simulink model "Model_TranslationEngine64"  (R2022b)
settings: Solver=FixedStepDiscrete  StartTime=0.0  StopTime=5  RelTol=1e-3  EnableMultiTasking=on
InitFcn:
  | % Initialize model
  | ModelSettings=BTConfig.GetModelSettings();
  | 
  | ModelSettings.Validate();
  | 
  | ModelInit;
  | 
  | 
  | % load library data
  | GainLibrary_data;
  | % Load saved values from partition process
  | CapturedConstMask.LoadMapFromFile(bdroot)
StartFcn:
  | % make sure all the simulated RTC requests are found
  | %RTC_SIM_OBJ.ValidateREQs();
undefined symbols (not defined in the file or in its folder): AA, BPLP, Column, NumHFRefBPF, NumHFRefLPF, NumMusicChannels, Row, VolumeMuteConfig
libraries: TuneVar x925, TOP x490, FeaturePath x111, CapturedConstLib x52
(part 32 of 34)

== matlab function Model_TranslationEngine64/ModelPreAmp/DecRate/Medusa5H1/MedusaHoligram/Medusa5H1 Part 3/On/Full-rate Mixer/Full-Rate Mixer with CAE & Fade Ramper/Fade Tuning/Downmix Weights Left/Trivial Translation ==
  data: TOP output size=[MedusaFRMConfig.LR_out MedusaFRMConfig.LR_in]; downmix_wts_Left input; MedusaFRMConfig parameter; TOP_CAE output size=[MedusaFRMConfig.LR_out MedusaFRMConfig.NumTailComp.LR]
  events: trigger input FUNCTION_CALL_EVENT
function [TOP,TOP_CAE]  = fcn(downmix_wts_Left, MedusaFRMConfig)
%#codegen
numLRIn = MedusaFRMConfig.LR_in;
NumCAEWeights = MedusaFRMConfig.NumTailComp.LR;

NumRows = MedusaFRMConfig.LR_out;
NumColumns = numLRIn + NumCAEWeights;
if(~ MedusaFRMConfig.includeCAE)
    NumColumns = numLRIn;
end

% Checks if the parameter satisfies dimensionality requirements
if(downmix_wts_Left.Size(1) ~= NumRows || downmix_wts_Left.Size(2) ~= NumColumns)
    TranslateError('The parameter ''medusa_frm_downmix_left'' must be a matrix consisting of %d rows and %d columns.', NumRows, NumColumns);
end

% Checks if the parameter values follow bound requirements
checkValues = (downmix_wts_Left.Value < 0);
if(sum(sum(checkValues)))          % Results in 0 if all values in the matrix respect the bound requirements
    TranslateError('The weights in ''medusa_frm_downmix_left'' must be greater than or equal to 0.');
end

% Assigning the parameter values to respective tuneTOPS
TOP = downmix_wts_Left.Value(:, 1:numLRIn);
if(~ MedusaFRMConfig.includeCAE)
    TOP_CAE = zeros(NumRows, NumCAEWeights);
else
    TOP_CAE = downmix_wts_Left.Value(:, numLRIn+1:end);
end

end

== matlab function Model_TranslationEngine64/ModelPreAmp/DecRate/Medusa5H1/MedusaHoligram/Medusa5H1 Part 3/On/Full-rate Mixer/Full-Rate Mixer with CAE & Fade Ramper/Fade Tuning/Downmix Weights Right/Trivial Translation ==
  data: TOP output size=[MedusaFRMConfig.LR_out MedusaFRMConfig.LR_in]; downmix_wts_Right input; MedusaFRMConfig parameter; TOP_CAE output size=[MedusaFRMConfig.LR_out MedusaFRMConfig.NumTailComp.LR]
  events: trigger input FUNCTION_CALL_EVENT
function [TOP,TOP_CAE]  = fcn(downmix_wts_Right, MedusaFRMConfig)
%#codegen
numLRIn = MedusaFRMConfig.LR_in;
NumCAEWeights = MedusaFRMConfig.NumTailComp.LR;

NumRows = MedusaFRMConfig.LR_out;
NumColumns = numLRIn + NumCAEWeights;
if(~ MedusaFRMConfig.includeCAE)
    NumColumns = numLRIn;
end

% Checks if the parameter satisfies dimensionality requirements
if(downmix_wts_Right.Size(1) ~= NumRows || downmix_wts_Right.Size(2) ~= NumColumns)
    TranslateError('The parameter ''medusa_frm_downmix_right'' must be a matrix consisting of %d rows and %d columns.', NumRows, NumColumns);
end

% Checks if the parameter values follow bound requirements
checkValues = (downmix_wts_Right.Value < 0);
if(sum(sum(checkValues)))          % Results in 0 if all values in the matrix respect the bound requirements
    TranslateError('The weights in ''medusa_frm_downmix_right'' must be greater than or equal to 0.');
end

% Assigning the parameter values to respective tuneTOPS
TOP = downmix_wts_Right.Value(:, 1:numLRIn);
if(~ MedusaFRMConfig.includeCAE)
    TOP_CAE = zeros(NumRows, NumCAEWeights);
else
    TOP_CAE = downmix_wts_Right.Value(:, numLRIn+1:end);
end

end

== matlab function Model_TranslationEngine64/ModelPreAmp/DecRate/Medusa5H1/MedusaHoligram/Medusa5H1 Part 3/On/Full-rate Mixer/Full-Rate Mixer with CAE & Fade Ramper/Fade Tuning/Forward Downmix Threshold/Trivial Translation ==
  data: TOP output; ForwardDownmixThreshold input
  events: trigger input FUNCTION_CALL_EVENT
function TOP  = fcn(ForwardDownmixThreshold)
%#codegen
% Checks if the parameter satisfies dimensionality requirements
if(numel(ForwardDownmixThreshold.Value) ~= 1)
   TranslateError('The parameter ''medusa_forward_downmix_threshold'' must be single dimensional.'); 
end

% Checks if the parameter value follows bound requirements
if((ForwardDownmixThreshold.Value < 0) || (ForwardDownmixThreshold.Value > 1))
   TranslateError('The value of ''medusa_forward_downmix_threshold'' must be between 0 and 1.'); 
end

TOP = ForwardDownmixThreshold.Value;

end

== matlab function Model_TranslationEngine64/ModelPreAmp/DecRate/Medusa5H1/MedusaHoligram/Medusa5H1 Part 3/On/Full-rate Mixer/Full-Rate Mixer with CAE & Fade Ramper/Fade Tuning/Foward Downmix Max/Trivial Translation ==
  data: TOP output; ForwardDownmixMax input
  events: trigger input FUNCTION_CALL_EVENT
function TOP  = fcn(ForwardDownmixMax)
%#codegen
% Checks if the parameter satisfies dimensionality requirements
if(numel(ForwardDownmixMax.Value) ~= 1)
   TranslateError('The parameter ''medusa_forward_downmix_max'' must be single dimensional.'); 
end

% Checks if the parameter value follows bound requirements
if((ForwardDownmixMax.Value < 0) || (ForwardDownmixMax.Value > 1))
   TranslateError('The value of ''medusa_forward_downmix_max'' must be between 0 and 1.'); 
end

TOP = ForwardDownmixMax.Value;

end

== matlab function Model_TranslationEngine64/ModelPreAmp/DecRate/AudioPilot35/Audiopilot_3_5/NoiseEstimationVariant/RegularNoiseEstimation/HFNoiseEstimatorCoh/PreProcessing/Bandpass or Lowpass Filter/InnerLink/PoolIirTunableWithReset/Translation ==
  data: RawSOS input; NumStages input; PoolNumStages output; PoolCoeffs output; MaxNumStages parameter; VariantUint8 parameter; NumChannels input
  events: trigger input FUNCTION_CALL_EVENT
function [PoolNumStages, PoolCoeffs] = pooliirTranslation(RawSOS, NumStages, MaxNumStages, VariantUint8,  NumChannels)
%#codegen

% Translation from raw SOS for pool SOS

% Some build time sanity size checking before calling the translation
if numel(NumStages.Value) ~= NumChannels
    error('Size of num stages has to match number of input channels')
end

if RawSOS.Size(2) ~= 6
    error ('Coefficient pool matrix must have 6 columns')
end

[PoolNumStages, PoolCoeffs] = poolIirTranslation(RawSOS, NumStages, MaxNumStages, VariantUint8);

% VariantStr = char(VariantUint8);
% switch (VariantStr)
%     case {"Generic","SharcPlusCore"}
%         % These variants order biquad coefficients in a compacted form
%         [PoolNumStages, PoolCoeffs] = pooliirTranslationFcn(RawSOS, NumStages, MaxNumStages);
%     case {"SharcPlusAccelGul","SharcPlusAccelGxp"}
%         % These variants order biquad coefficients for the ADI accelerator
%         [PoolNumStages, PoolCoeffs] = pooliirAccelTranslationFcn(RawSOS, NumStages, MaxNumStages);
%     case{"Hexagon"}
%         % Hexagon specific order for biquad coefficients 
%         [PoolNumStages, PoolCoeffs] = PoolIirHexagonTranslationFcn(RawSOS, NumStages, MaxNumStages);
%     case{"ArmNeonV7V8"}
%         [PoolNumStages, PoolCoeffs] = PoolIirArmNeonV7V8TranslationFcn(RawSOS, NumStages, MaxNumStages);
%     otherwise
%         % This is a build-time error, not a translation error. The
%         % selected build-time variant is not supported for translation
%         error('Invalid implementation type: [%s]', VariantStr);
% end

end

== matlab function Model_TranslationEngine64/ModelPreAmp/DecRate/Medusa5H1/MedusaHoligram/Medusa5H1 Part 3/On/Full-rate Mixer/Full-Rate Mixer with CAE & Fade Ramper/SLC Tuning/Detent Level CS/Trivial Translation ==
  data: TOP output size=[MedusaFRMConfig.CS_out MedusaFRMConfig.CS_in]; detentGain_CS input; MedusaFRMConfig parameter; TOP_CAE output size=[MedusaFRMConfig.CS_out MedusaFRMConfig.NumTailComp.CS]
  events: trigger input FUNCTION_CALL_EVENT
function [TOP, TOP_CAE]  = fcn(detentGain_CS, MedusaFRMConfig)
%#codegen
numCSIn = MedusaFRMConfig.CS_in;
NumCAEWeights = MedusaFRMConfig.NumTailComp.CS;

NumRows = MedusaFRMConfig.CS_out;
NumColumns = numCSIn + NumCAEWeights;
if(~ MedusaFRMConfig.includeCAE)
    NumColumns = numCSIn;
end

% Checks if the parameter satisfies dimensionality requirements
if(detentGain_CS.Size(1) ~= NumRows || detentGain_CS.Size(2) ~= NumColumns)
    TranslateError('The parameter ''medusa_frm_cs_detent'' must be a matrix consisting of %d rows and %d columns.', NumRows, NumColumns);
end

% Checks if the parameter values follow bound requirements
checkValues = (detentGain_CS.Value < 0);    
if(sum(sum(checkValues)))       % Results in 0 if all values in the matrix respect the bound requirements
    TranslateError('The weights in ''medusa_frm_cs_detent'' must be greater than or equal to 0.');
end

% Assigning the parameter values to respective tuneTOPS
TOP = detentGain_CS.Value(:, 1:numCSIn);
if(~ MedusaFRMConfig.includeCAE)
    TOP_CAE = zeros(NumRows, NumCAEWeights);
else
    TOP_CAE = detentGain_CS.Value(:, numCSIn+1:end);
end

end

== matlab function Model_TranslationEngine64/ModelPreAmp/DecRate/Medusa5H1/MedusaHoligram/Medusa5H1 Part 3/On/Full-rate Mixer/Full-Rate Mixer with CAE & Fade Ramper/SLC Tuning/Detent Level Left/Trivial Translation ==
  data: TOP output size=[MedusaFRMConfig.LR_out MedusaFRMConfig.LR_in]; detentGain_Left input; MedusaFRMConfig parameter; TOP_CAE output size=[MedusaFRMConfig.LR_out MedusaFRMConfig.NumTailComp.LR]
  events: trigger input FUNCTION_CALL_EVENT
function [TOP, TOP_CAE]  = fcn(detentGain_Left, MedusaFRMConfig)
%#codegen
numLRIn = MedusaFRMConfig.LR_in;
NumCAEWeights = MedusaFRMConfig.NumTailComp.LR;

NumRows = MedusaFRMConfig.LR_out;
NumColumns = numLRIn + NumCAEWeights;
if(~ MedusaFRMConfig.includeCAE)
    NumColumns = numLRIn;
end

% Checks if the parameter satisfies dimensionality requirements
if(detentGain_Left.Size(1) ~= NumRows || detentGain_Left.Size(2) ~= NumColumns)
    TranslateError('The parameter ''medusa_frm_left_detent'' must be a matrix consisting of %d rows and %d columns.', NumRows, NumColumns);
end

% Checks if the parameter values follow bound requirements
checkValues = (detentGain_Left.Value < 0);    
if(sum(sum(checkValues)))       % Results in 0 if all values in the matrix respect the bound requirements
    TranslateError('The weights in ''medusa_frm_left_detent'' must be greater than or equal to 0.');
end

% Assigning the parameter values to respective tuneTOPS
TOP = detentGain_Left.Value(:, 1:numLRIn);
if(~ MedusaFRMConfig.includeCAE)
    TOP_CAE = zeros(NumRows, NumCAEWeights);
else
    TOP_CAE = detentGain_Left.Value(:, numLRIn+1:end);
end

end

== matlab function Model_TranslationEngine64/ModelPreAmp/DecRate/Medusa5H1/MedusaHoligram/Medusa5H1 Part 3/On/Full-rate Mixer/Full-Rate Mixer with CAE & Fade Ramper/SLC Tuning/Detent Level Right/Trivial Translation ==
  data: TOP output size=[MedusaFRMConfig.LR_out MedusaFRMConfig.LR_in]; detentGain_Right input; MedusaFRMConfig parameter; TOP_CAE output size=[MedusaFRMConfig.LR_out MedusaFRMConfig.NumTailComp.LR]
  events: trigger input FUNCTION_CALL_EVENT
function [TOP, TOP_CAE]  = fcn(detentGain_Right, MedusaFRMConfig)
%#codegen
numLRIn = MedusaFRMConfig.LR_in;
NumCAEWeights = MedusaFRMConfig.NumTailComp.LR;

NumRows = MedusaFRMConfig.LR_out;
NumColumns = numLRIn + NumCAEWeights;
if(~ MedusaFRMConfig.includeCAE)
    NumColumns = numLRIn;
end

% Checks if the parameter satisfies dimensionality requirements
if(detentGain_Right.Size(1) ~= NumRows || detentGain_Right.Size(2) ~= NumColumns)
    TranslateError('The parameter ''medusa_frm_right_detent'' must be a matrix consisting of %d rows and %d columns.', NumRows, NumColumns);
end

% Checks if the parameter values follow bound requirements
checkValues = (detentGain_Right.Value < 0);    
if(sum(sum(checkValues)))       % Results in 0 if all values in the matrix respect the bound requirements
    TranslateError('The weights in ''medusa_frm_right_detent'' must be greater than or equal to 0.');
end

% Assigning the parameter values to respective tuneTOPS
TOP = detentGain_Right.Value(:, 1:numLRIn);
if(~ MedusaFRMConfig.includeCAE)
    TOP_CAE = zeros(NumRows, NumCAEWeights);
else
    TOP_CAE = detentGain_Right.Value(:, numLRIn+1:end);
end

end

== matlab function Model_TranslationEngine64/ModelPreAmp/DecRate/Medusa5H1/MedusaHoligram/Medusa5H1 Part 3/On/Full-rate Mixer/Full-Rate Mixer with CAE & Fade Ramper/SLC Tuning/Interpolation Method/Trivial Translation ==
  data: TOP output; interpolationMethod input
  events: trigger input FUNCTION_CALL_EVENT
function TOP  = fcn(interpolationMethod)
%#codegen
% Checks if the parameter satisfies dimensionality requirements
if(numel(interpolationMethod.Value) ~= 1)
   TranslateError('The parameter ''medusa_surround_db_interpolation'' must be single dimensional.'); 
end

% Checks if the parameter value follows bound requirements
if((interpolationMethod.Value ~= 0) && (interpolationMethod.Value ~= 1))
   TranslateError('The value of ''medusa_surround_db_interpolation'' must be either 0 (for linear interpolation) or 1 (for dB-linear interpolation).'); 
end

TOP = interpolationMethod.Value;

end

== matlab function Model_TranslationEngine64/ModelPreAmp/DecRate/Medusa5H1/MedusaHoligram/Medusa5H1 Part 3/On/Full-rate Mixer/Full-Rate Mixer with CAE & Fade Ramper/SLC Tuning/Max Level CS/Trivial Translation ==
  data: TOP output size=[MedusaFRMConfig.CS_out MedusaFRMConfig.CS_in]; maxGain_CS input; MedusaFRMConfig parameter; TOP_CAE output size=[MedusaFRMConfig.CS_out MedusaFRMConfig.NumTailComp.CS]
  events: trigger input FUNCTION_CALL_EVENT
function [TOP, TOP_CAE] = fcn(maxGain_CS, MedusaFRMConfig)
%#codegen
numCSIn = MedusaFRMConfig.CS_in;
NumCAEWeights = MedusaFRMConfig.NumTailComp.CS;

NumRows = MedusaFRMConfig.CS_out;
NumColumns = numCSIn + NumCAEWeights;
if(~ MedusaFRMConfig.includeCAE)
    NumColumns = numCSIn;
end

% Checks if the parameter satisfies dimensionality requirements
if(maxGain_CS.Size(1) ~= NumRows || maxGain_CS.Size(2) ~= NumColumns)
    TranslateError('The parameter ''medusa_frm_cs_max'' must be a matrix consisting of %d rows and %d columns.', NumRows, NumColumns);
end

% Checks if the parameter values follow bound requirements
checkValues = (maxGain_CS.Value < 0);
if(sum(sum(checkValues)))          % Results in 0 if all values in the matrix respect the bound requirements
    TranslateError('The weights in ''medusa_frm_cs_max'' must be greater than or equal to 0.');
end

% Assigning the parameter values to respective tuneTOPS
TOP = maxGain_CS.Value(:, 1:numCSIn);
if(~ MedusaFRMConfig.includeCAE)
    TOP_CAE = zeros(NumRows, NumCAEWeights);
else
    TOP_CAE = maxGain_CS.Value(:, numCSIn+1:end);
end

end

== matlab function Model_TranslationEngine64/ModelPreAmp/DecRate/Medusa5H1/MedusaHoligram/Medusa5H1 Part 3/On/Full-rate Mixer/Full-Rate Mixer with CAE & Fade Ramper/SLC Tuning/Max Level Left/Trivial Translation ==
  data: TOP output size=[MedusaFRMConfig.LR_out MedusaFRMConfig.LR_in]; maxGain_Left input; MedusaFRMConfig parameter; TOP_CAE output size=[MedusaFRMConfig.LR_out MedusaFRMConfig.NumTailComp.LR]
  events: trigger input FUNCTION_CALL_EVENT
function [TOP, TOP_CAE]  = fcn(maxGain_Left, MedusaFRMConfig)
%#codegen
numLRIn = MedusaFRMConfig.LR_in;
NumCAEWeights = MedusaFRMConfig.NumTailComp.LR;

NumRows = MedusaFRMConfig.LR_out;
NumColumns = numLRIn + NumCAEWeights;
if(~ MedusaFRMConfig.includeCAE)
    NumColumns = numLRIn;
end

% Checks if the parameter satisfies dimensionality requirements
if(maxGain_Left.Size(1) ~= NumRows || maxGain_Left.Size(2) ~= NumColumns)
    TranslateError('The parameter ''medusa_frm_left_max'' must be a matrix consisting of %d rows and %d columns.', NumRows, NumColumns);
end

% Checks if the parameter values follow bound requirements
checkValues = (maxGain_Left.Value < 0);
if(sum(sum(checkValues)))          % Results in 0 if all values in the matrix respect the bound requirements
    TranslateError('The weights in ''medusa_frm_left_max'' must be greater than or equal to 0.');
end

% Assigning the parameter values to respective tuneTOPS
TOP = maxGain_Left.Value(:, 1:numLRIn);
if(~ MedusaFRMConfig.includeCAE)
    TOP_CAE = zeros(NumRows, NumCAEWeights);
else
    TOP_CAE = maxGain_Left.Value(:, numLRIn+1:end);
end

end

== matlab function Model_TranslationEngine64/ModelPreAmp/DecRate/Medusa5H1/MedusaHoligram/Medusa5H1 Part 3/On/Full-rate Mixer/Full-Rate Mixer with CAE & Fade Ramper/SLC Tuning/Max Level Right/Trivial Translation ==
  data: TOP output size=[MedusaFRMConfig.LR_out MedusaFRMConfig.LR_in]; maxGain_Right input; MedusaFRMConfig parameter; TOP_CAE output size=[MedusaFRMConfig.LR_out MedusaFRMConfig.NumTailComp.LR]
  events: trigger input FUNCTION_CALL_EVENT
function [TOP, TOP_CAE]  = fcn(maxGain_Right, MedusaFRMConfig)
%#codegen
numLRIn = MedusaFRMConfig.LR_in;
NumCAEWeights = MedusaFRMConfig.NumTailComp.LR;

NumRows = MedusaFRMConfig.LR_out;
NumColumns = numLRIn + NumCAEWeights;
if(~ MedusaFRMConfig.includeCAE)
    NumColumns = numLRIn;
end

% Checks if the parameter satisfies dimensionality requirements
if(maxGain_Right.Size(1) ~= NumRows || maxGain_Right.Size(2) ~= NumColumns)
    TranslateError('The parameter ''medusa_frm_right_max'' must be a matrix consisting of %d rows and %d columns.', NumRows, NumColumns);
end

% Checks if the parameter values follow bound requirements
checkValues = (maxGain_Right.Value < 0);
if(sum(sum(checkValues)))          % Results in 0 if all values in the matrix respect the bound requirements
    TranslateError('The weights in ''medusa_frm_right_max'' must be greater than or equal to 0.');
end

% Assigning the parameter values to respective tuneTOPS
TOP = maxGain_Right.Value(:, 1:numLRIn);
if(~ MedusaFRMConfig.includeCAE)
    TOP_CAE = zeros(NumRows, NumCAEWeights);
else
    TOP_CAE = maxGain_Right.Value(:, numLRIn+1:end);
end

end

== matlab function Model_TranslationEngine64/ModelPreAmp/DecRate/Medusa5H1/MedusaHoligram/Medusa5H1 Part 3/On/Full-rate Mixer/Full-Rate Mixer with CAE & Fade Ramper/SLC Tuning/Min Level CS/Trivial Translation ==
  data: TOP output size=[MedusaFRMConfig.CS_out MedusaFRMConfig.CS_in]; minGain_CS input; MedusaFRMConfig parameter; TOP_CAE output size=[MedusaFRMConfig.CS_out MedusaFRMConfig.NumTailComp.CS]
  events: trigger input FUNCTION_CALL_EVENT
function [TOP, TOP_CAE]  = fcn(minGain_CS, MedusaFRMConfig)
%#codegen
numCSIn = MedusaFRMConfig.CS_in;
NumCAEWeights = MedusaFRMConfig.NumTailComp.CS;

NumRows = MedusaFRMConfig.CS_out;
NumColumns = numCSIn + NumCAEWeights;
if(~ MedusaFRMConfig.includeCAE)
    NumColumns = numCSIn;
end

% Checks if the parameter satisfies dimensionality requirements
if(minGain_CS.Size(1) ~= NumRows || minGain_CS.Size(2) ~= NumColumns)
    TranslateError('The parameter ''medusa_frm_cs_min'' must be a matrix consisting of %d rows and %d columns.', NumRows, NumColumns);
end

% Checks if the parameter values follow bound requirements
checkValues = (minGain_CS.Value < 0);
if(sum(sum(checkValues)))          % Results in 0 if all values in the matrix respect the bound requirements
    TranslateError('The weights in ''medusa_frm_cs_min'' must be greater than or equal to 0.');
end

% Assigning the parameter values to respective tuneTOPS
TOP = minGain_CS.Value(:, 1:numCSIn);
if(~ MedusaFRMConfig.includeCAE)
    TOP_CAE = zeros(NumRows, NumCAEWeights);
else
    TOP_CAE = minGain_CS.Value(:, numCSIn+1:end);
end

end

== matlab function Model_TranslationEngine64/ModelPreAmp/DecRate/Medusa5H1/MedusaHoligram/Medusa5H1 Part 3/On/Full-rate Mixer/Full-Rate Mixer with CAE & Fade Ramper/SLC Tuning/Min Level Left/Trivial Translation ==
  data: TOP output size=[MedusaFRMConfig.LR_out MedusaFRMConfig.LR_in]; minGain_Left input; MedusaFRMConfig parameter; TOP_CAE output size=[MedusaFRMConfig.LR_out MedusaFRMConfig.NumTailComp.LR]
  events: trigger input FUNCTION_CALL_EVENT
function [TOP, TOP_CAE]  = fcn(minGain_Left, MedusaFRMConfig)
%#codegen
numLRIn = MedusaFRMConfig.LR_in;
NumCAEWeights = MedusaFRMConfig.NumTailComp.LR;

NumRows = MedusaFRMConfig.LR_out;
NumColumns = numLRIn + NumCAEWeights;
if(~ MedusaFRMConfig.includeCAE)
    NumColumns = numLRIn;
end

% Checks if the parameter satisfies dimensionality requirements
if(minGain_Left.Size(1) ~= NumRows || minGain_Left.Size(2) ~= NumColumns)
    TranslateError('The parameter ''medusa_frm_left_min'' must be a matrix consisting of %d rows and %d columns.', NumRows, NumColumns);
end

% Checks if the parameter values follow bound requirements
checkValues = (minGain_Left.Value < 0);
if(sum(sum(checkValues)))          % Results in 0 if all values in the matrix respect the bound requirements
    TranslateError('The weights in ''medusa_frm_left_min'' must be greater than or equal to 0.');
end

% Assigning the parameter values to respective tuneTOPS
TOP = minGain_Left.Value(:, 1:numLRIn);
if(~ MedusaFRMConfig.includeCAE)
    TOP_CAE = zeros(NumRows, NumCAEWeights);
else
    TOP_CAE = minGain_Left.Value(:, numLRIn+1:end);
end

end

== matlab function Model_TranslationEngine64/ModelPreAmp/DecRate/Medusa5H1/MedusaHoligram/Medusa5H1 Part 3/On/Full-rate Mixer/Full-Rate Mixer with CAE & Fade Ramper/SLC Tuning/Min Level Right/Trivial Translation ==
  data: TOP output size=[MedusaFRMConfig.LR_out MedusaFRMConfig.LR_in]; minGain_Right input; MedusaFRMConfig parameter; TOP_CAE output size=[MedusaFRMConfig.LR_out MedusaFRMConfig.NumTailComp.LR]
  events: trigger input FUNCTION_CALL_EVENT
function [TOP, TOP_CAE]  = fcn(minGain_Right, MedusaFRMConfig)
%#codegen
numLRIn = MedusaFRMConfig.LR_in;
NumCAEWeights = MedusaFRMConfig.NumTailComp.LR;

NumRows = MedusaFRMConfig.LR_out;
NumColumns = numLRIn + NumCAEWeights;
if(~ MedusaFRMConfig.includeCAE)
    NumColumns = numLRIn;
end

% Checks if the parameter satisfies dimensionality requirements
if(minGain_Right.Size(1) ~= NumRows || minGain_Right.Size(2) ~= NumColumns)
    TranslateError('The parameter ''medusa_frm_right_min'' must be a matrix consisting of %d rows and %d columns.', NumRows, NumColumns);
end

% Checks if the parameter values follow bound requirements
checkValues = (minGain_Right.Value < 0);
if(sum(sum(checkValues)))          % Results in 0 if all values in the matrix respect the bound requirements
    TranslateError('The weights in ''medusa_frm_right_min'' must be greater than or equal to 0.');
end

% Assigning the parameter values to respective tuneTOPS
TOP = minGain_Right.Value(:, 1:numLRIn);
if(~ MedusaFRMConfig.includeCAE)
    TOP_CAE = zeros(NumRows, NumCAEWeights);
else
    TOP_CAE = minGain_Right.Value(:, numLRIn+1:end);
end

end

== matlab function Model_TranslationEngine64/ModelPreAmp/DecRate/Medusa5H1/MedusaHoligram/Medusa5H1 Part 3/On/Premix/Premix with Mono-Surround & CAE with Fade Ramper/CS Processing/MS Tune/translation ==
  data: phi output; PhaseAngle input; cos_phi output; sin_phi output
  events: trigger input FUNCTION_CALL_EVENT
function [phi, cos_phi, sin_phi]  = fcn(PhaseAngle)
%#codegen
% Checks if the parameter satisfies dimensionality requirements
if(numel(PhaseAngle.Value) ~= 1)
   TranslateError('The parameter ''medusa_mono_c_s_blending_angle_deg'' must be single dimensional.'); 
end

% Checks if the parameter value follows bound requirements
if((PhaseAngle.Value < 0) || (PhaseAngle.Value >= 360))
   TranslateError('The value of ''medusa_mono_c_s_blending_angle_deg'' must be in degrees and can range from 0 to 359.'); 
end

phi = PhaseAngle.Value;
cos_phi = cosd(phi);
sin_phi = sind(phi);

end

== matlab function Model_TranslationEngine64/ModelPreAmp/DecRate/Medusa5H1/MedusaHoligram/Medusa5H1 Part 3/On/Premix/Premix with Mono-Surround & CAE with Fade Ramper/Fade Tuning/Backward Downmix Max/Trivial Translation ==
  data: TOP output; BackwardDownmixMax input
  events: trigger input FUNCTION_CALL_EVENT
function TOP  = fcn(BackwardDownmixMax)
%#codegen
% Checks if the parameter satisfies dimensionality requirements
if(numel(BackwardDownmixMax.Value) ~= 1)
   TranslateError('The parameter ''medusa_backward_downmix_max'' must be single dimensional.'); 
end

% Checks if the parameter value follows bound requirements
if((BackwardDownmixMax.Value < 0) || (BackwardDownmixMax.Value > 1))
   TranslateError('The value of ''medusa_backward_downmix_max'' must be between 0 and 1.'); 
end

TOP = BackwardDownmixMax.Value;

end

== matlab function Model_TranslationEngine64/ModelPreAmp/DecRate/Medusa5H1/MedusaHoligram/Medusa5H1 Part 3/On/Premix/Premix with Mono-Surround & CAE with Fade Ramper/Fade Tuning/Backward Downmix Threshold/Trivial Translation ==
  data: TOP output; BackwardDownmixThreshold input
  events: trigger input FUNCTION_CALL_EVENT
function TOP  = fcn(BackwardDownmixThreshold)
%#codegen
% Checks if the parameter satisfies dimensionality requirements
if(numel(BackwardDownmixThreshold.Value) ~= 1)
   TranslateError('The parameter ''medusa_backward_downmix_threshold'' must be single dimensional.'); 
end

% Checks if the parameter value follows bound requirements
if((BackwardDownmixThreshold.Value < 0) || (BackwardDownmixThreshold.Value > 1))
   TranslateError('The value of ''medusa_backward_downmix_threshold'' must be between 0 and 1.'); 
end

TOP = BackwardDownmixThreshold.Value;

end

== matlab function Model_TranslationEngine64/ModelPreAmp/DecRate/Medusa5H1/MedusaHoligram/Medusa5H1 Part 3/On/Premix/Premix with Mono-Surround & CAE with Fade Ramper/Fade Tuning/Downmix Weights CS/Trivial Translation ==
  data: TOP output size=[MedusaPremixConfig.CS_out MedusaPremixConfig.CS_in]; downmix_wts_CS input; MedusaPremixConfig parameter; TOP_CAE output size=[MedusaPremixConfig.CS_out MedusaPremixConfig.NumTailComp.CS]
  events: trigger input FUNCTION_CALL_EVENT
function [TOP,TOP_CAE]  = fcn(downmix_wts_CS, MedusaPremixConfig)
%#codegen
numCSIn = MedusaPremixConfig.CS_in;
NumCAEWeights = MedusaPremixConfig.NumTailComp.CS;

NumRows = MedusaPremixConfig.CS_out;
NumColumns = numCSIn + NumCAEWeights;
if(~ MedusaPremixConfig.includeCAE)
    NumColumns = numCSIn;
end

% Checks if the parameter satisfies dimensionality requirements
if(downmix_wts_CS.Size(1) ~= NumRows || downmix_wts_CS.Size(2) ~= NumColumns)
    TranslateError('The parameter ''medusa_premix_downmix_cs'' must be a matrix consisting of %d rows and %d columns.', NumRows, NumColumns);
end

% Checks if the parameter values follow bound requirements
checkValues = (downmix_wts_CS.Value < 0);
if(sum(sum(checkValues)))          % Results in 0 if all values in the matrix respect the bound requirements
    TranslateError('The weights in ''medusa_premix_downmix_CS'' must be greater than or equal to 0.');
end

% Assigning the parameter values to respective tuneTOPS
TOP = downmix_wts_CS.Value(:, 1:numCSIn);
if(~ MedusaPremixConfig.includeCAE)
    TOP_CAE = zeros(NumRows, NumCAEWeights);
else
    TOP_CAE = downmix_wts_CS.Value(:, numCSIn+1:end);
end

end

== matlab function Model_TranslationEngine64/ModelPreAmp/DecRate/AudioPilot35/Audiopilot_3_5/GainCalculation/BoostMapAdjustment/AudiopilotOn/Treble0Enable ==
  data: on input; slopeOut output; slope input
  events: trigger input FUNCTION_CALL_EVENT
function slopeOut  = enable(on,slope)
%#codegen
slopeOut = slope.Value * on.Value;

== matlab function Model_TranslationEngine64/ModelPreAmp/DecRate/Medusa5H1/MedusaHoligram/Medusa5H1 Part 3/On/Premix/Premix with Mono-Surround & CAE with Fade Ramper/Fade Tuning/Downmix Weights Left/Trivial Translation ==
  data: TOP output size=[MedusaPremixConfig.LR_out MedusaPremixConfig.LR_in]; downmix_wts_Left input; MedusaPremixConfig parameter; TOP_CAE output size=[MedusaPremixConfig.LR_out MedusaPremixConfig.NumTailComp.LR]
  events: trigger input FUNCTION_CALL_EVENT
function [TOP,TOP_CAE]  = fcn(downmix_wts_Left, MedusaPremixConfig)
%#codegen
numLRIn = MedusaPremixConfig.LR_in;
NumCAEWeights = MedusaPremixConfig.NumTailComp.LR;

NumRows = MedusaPremixConfig.LR_out;
NumColumns = numLRIn + NumCAEWeights;
if(~ MedusaPremixConfig.includeCAE)
    NumColumns = numLRIn;
end

% Checks if the parameter satisfies dimensionality requirements
if(downmix_wts_Left.Size(1) ~= NumRows || downmix_wts_Left.Size(2) ~= NumColumns)
    TranslateError('The parameter ''medusa_premix_downmix_left'' must be a matrix consisting of %d rows and %d columns.', NumRows, NumColumns);
end

% Checks if the parameter values follow bound requirements
checkValues = (downmix_wts_Left.Value < 0);
if(sum(sum(checkValues)))          % Results in 0 if all values in the matrix respect the bound requirements
    TranslateError('The weights in ''medusa_premix_downmix_left'' must be greater than or equal to 0.');
end

% Assigning the parameter values to respective tuneTOPS
TOP = downmix_wts_Left.Value(:, 1:numLRIn);
if(~ MedusaPremixConfig.includeCAE)
    TOP_CAE = zeros(NumRows, NumCAEWeights);
else
    TOP_CAE = downmix_wts_Left.Value(:, numLRIn+1:end);
end

end

== matlab function Model_TranslationEngine64/ModelPreAmp/DecRate/Medusa5H1/MedusaHoligram/Medusa5H1 Part 3/On/Premix/Premix with Mono-Surround & CAE with Fade Ramper/Fade Tuning/Downmix Weights Right/Trivial Translation ==
  data: TOP output size=[MedusaPremixConfig.LR_out MedusaPremixConfig.LR_in]; downmix_wts_Right input; MedusaPremixConfig parameter; TOP_CAE output size=[MedusaPremixConfig.LR_out MedusaPremixConfig.NumTailComp.LR]
  events: trigger input FUNCTION_CALL_EVENT
function [TOP,TOP_CAE]  = fcn(downmix_wts_Right, MedusaPremixConfig)
%#codegen
numLRIn = MedusaPremixConfig.LR_in;
NumCAEWeights = MedusaPremixConfig.NumTailComp.LR;

NumRows = MedusaPremixConfig.LR_out;
NumColumns = numLRIn + NumCAEWeights;
if(~ MedusaPremixConfig.includeCAE)
    NumColumns = numLRIn;
end

% Checks if the parameter satisfies dimensionality requirements
if(downmix_wts_Right.Size(1) ~= NumRows || downmix_wts_Right.Size(2) ~= NumColumns)
    TranslateError('The parameter ''medusa_premix_downmix_right'' must be a matrix consisting of %d rows and %d columns.', NumRows, NumColumns);
end

% Checks if the parameter values follow bound requirements
checkValues = (downmix_wts_Right.Value < 0);
if(sum(sum(checkValues)))          % Results in 0 if all values in the matrix respect the bound requirements
    TranslateError('The weights in ''medusa_premix_downmix_right'' must be greater than or equal to 0.');
end

% Assigning the parameter values to respective tuneTOPS
TOP = downmix_wts_Right.Value(:, 1:numLRIn);
if(~ MedusaPremixConfig.includeCAE)
    TOP_CAE = zeros(NumRows, NumCAEWeights);
else
    TOP_CAE = downmix_wts_Right.Value(:, numLRIn+1:end);
end

end

== matlab function Model_TranslationEngine64/ModelPreAmp/DecRate/Medusa5H1/MedusaHoligram/Medusa5H1 Part 3/On/Premix/Premix with Mono-Surround & CAE with Fade Ramper/Fade Tuning/Forward Downmix Threshold/Trivial Translation ==
  data: TOP output; ForwardDownmixThreshold input
  events: trigger input FUNCTION_CALL_EVENT
function TOP  = fcn(ForwardDownmixThreshold)
%#codegen
% Checks if the parameter satisfies dimensionality requirements
if(numel(ForwardDownmixThreshold.Value) ~= 1)
   TranslateError('The parameter ''medusa_forward_downmix_threshold'' must be single dimensional.'); 
end

% Checks if the parameter value follows bound requirements
if((ForwardDownmixThreshold.Value < 0) || (ForwardDownmixThreshold.Value > 1))
   TranslateError('The value of ''medusa_forward_downmix_threshold'' must be between 0 and 1.'); 
end

TOP = ForwardDownmixThreshold.Value;

end

== matlab function Model_TranslationEngine64/ModelPreAmp/DecRate/Medusa5H1/MedusaHoligram/Medusa5H1 Part 3/On/Premix/Premix with Mono-Surround & CAE with Fade Ramper/Fade Tuning/Foward Downmix Max/Trivial Translation ==
  data: TOP output; ForwardDownmixMax input
  events: trigger input FUNCTION_CALL_EVENT
function TOP  = fcn(ForwardDownmixMax)
%#codegen
% Checks if the parameter satisfies dimensionality requirements
if(numel(ForwardDownmixMax.Value) ~= 1)
   TranslateError('The parameter ''medusa_forward_downmix_max'' must be single dimensional.'); 
end

% Checks if the parameter value follows bound requirements
if((ForwardDownmixMax.Value < 0) || (ForwardDownmixMax.Value > 1))
   TranslateError('The value of ''medusa_forward_downmix_max'' must be between 0 and 1.'); 
end

TOP = ForwardDownmixMax.Value;

end

== matlab function Model_TranslationEngine64/ModelPreAmp/DecRate/Medusa5H1/MedusaHoligram/Medusa5H1 Part 3/On/Premix/Premix with Mono-Surround & CAE with Fade Ramper/SLC Tuning/Detent Level CS/Trivial Translation ==
  data: TOP output size=[MedusaPremixConfig.CS_out MedusaPremixConfig.CS_in]; detentGain_CS input; MedusaPremixConfig parameter; TOP_CAE output size=[MedusaPremixConfig.CS_out MedusaPremixConfig.NumTailComp.CS]
  events: trigger input FUNCTION_CALL_EVENT
function [TOP, TOP_CAE]  = fcn(detentGain_CS, MedusaPremixConfig)
%#codegen
numCSIn = MedusaPremixConfig.CS_in;
NumCAEWeights = MedusaPremixConfig.NumTailComp.CS;

NumRows = MedusaPremixConfig.CS_out;
NumColumns = numCSIn + NumCAEWeights;
if(~ MedusaPremixConfig.includeCAE)
    NumColumns = numCSIn;
end

% Checks if the parameter satisfies dimensionality requirements
if(detentGain_CS.Size(1) ~= NumRows || detentGain_CS.Size(2) ~= NumColumns)
    TranslateError('The parameter ''medusa_premix_cs_detent'' must be a matrix consisting of %d rows and %d columns.', NumRows, NumColumns);
end

% Checks if the parameter values follow bound requirements
checkValues = (detentGain_CS.Value < 0);    
if(sum(sum(checkValues)))       % Results in 0 if all values in the matrix respect the bound requirements
    TranslateError('The weights in ''medusa_premix_cs_detent'' must be greater than or equal to 0.');
end

% Assigning the parameter values to respective tuneTOPS
TOP = detentGain_CS.Value(:, 1:numCSIn);
if(~ MedusaPremixConfig.includeCAE)
    TOP_CAE = zeros(NumRows, NumCAEWeights);
else
    TOP_CAE = detentGain_CS.Value(:, numCSIn+1:end);
end

end

== matlab function Model_TranslationEngine64/ModelPreAmp/DecRate/Medusa5H1/MedusaHoligram/Medusa5H1 Part 3/On/Premix/Premix with Mono-Surround & CAE with Fade Ramper/SLC Tuning/Detent Level Left/Trivial Translation ==
  data: TOP output size=[MedusaPremixConfig.LR_out MedusaPremixConfig.LR_in]; detentGain_Left input; MedusaPremixConfig parameter; TOP_CAE output size=[MedusaPremixConfig.LR_out MedusaPremixConfig.NumTailComp.LR]
  events: trigger input FUNCTION_CALL_EVENT
function [TOP, TOP_CAE]  = fcn(detentGain_Left, MedusaPremixConfig)
%#codegen
numLRIn = MedusaPremixConfig.LR_in;
NumCAEWeights = MedusaPremixConfig.NumTailComp.LR;

NumRows = MedusaPremixConfig.LR_out;
NumColumns = numLRIn + NumCAEWeights;
if(~ MedusaPremixConfig.includeCAE)
    NumColumns = numLRIn;
end

% Checks if the parameter satisfies dimensionality requirements
if(detentGain_Left.Size(1) ~= NumRows || detentGain_Left.Size(2) ~= NumColumns)
    TranslateError('The parameter ''medusa_premix_left_detent'' must be a matrix consisting of %d rows and %d columns.', NumRows, NumColumns);
end

% Checks if the parameter values follow bound requirements
checkValues = (detentGain_Left.Value < 0);    
if(sum(sum(checkValues)))       % Results in 0 if all values in the matrix respect the bound requirements
    TranslateError('The weights in ''medusa_premix_left_detent'' must be greater than or equal to 0.');
end

% Assigning the parameter values to respective tuneTOPS
TOP = detentGain_Left.Value(:, 1:numLRIn);
if(~ MedusaPremixConfig.includeCAE)
    TOP_CAE = zeros(NumRows, NumCAEWeights);
else
    TOP_CAE = detentGain_Left.Value(:, numLRIn+1:end);
end

end

== matlab function Model_TranslationEngine64/ModelPreAmp/DecRate/Medusa5H1/MedusaHoligram/Medusa5H1 Part 3/On/Premix/Premix with Mono-Surround & CAE with Fade Ramper/SLC Tuning/Detent Level Right/Trivial Translation ==
  data: TOP output size=[MedusaPremixConfig.LR_out MedusaPremixConfig.LR_in]; detentGain_Right input; MedusaPremixConfig parameter; TOP_CAE output size=[MedusaPremixConfig.LR_out MedusaPremixConfig.NumTailComp.LR]
  events: trigger input FUNCTION_CALL_EVENT
function [TOP, TOP_CAE]  = fcn(detentGain_Right, MedusaPremixConfig)
%#codegen
numLRIn = MedusaPremixConfig.LR_in;
NumCAEWeights = MedusaPremixConfig.NumTailComp.LR;

NumRows = MedusaPremixConfig.LR_out;
NumColumns = numLRIn + NumCAEWeights;
if(~ MedusaPremixConfig.includeCAE)
    NumColumns = numLRIn;
end

% Checks if the parameter satisfies dimensionality requirements
if(detentGain_Right.Size(1) ~= NumRows || detentGain_Right.Size(2) ~= NumColumns)
    TranslateError('The parameter ''medusa_premix_right_detent'' must be a matrix consisting of %d rows and %d columns.', NumRows, NumColumns);
end

% Checks if the parameter values follow bound requirements
checkValues = (detentGain_Right.Value < 0);    
if(sum(sum(checkValues)))       % Results in 0 if all values in the matrix respect the bound requirements
    TranslateError('The weights in ''medusa_premix_right_detent'' must be greater than or equal to 0.');
end

% Assigning the parameter values to respective tuneTOPS
TOP = detentGain_Right.Value(:, 1:numLRIn);
if(~ MedusaPremixConfig.includeCAE)
    TOP_CAE = zeros(NumRows, NumCAEWeights);
else
    TOP_CAE = detentGain_Right.Value(:, numLRIn+1:end);
end

end

== matlab function Model_TranslationEngine64/ModelPreAmp/DecRate/Medusa5H1/MedusaHoligram/Medusa5H1 Part 3/On/Premix/Premix with Mono-Surround & CAE with Fade Ramper/SLC Tuning/Interpolation Method/Trivial Translation ==
  data: TOP output; interpolationMethod input
  events: trigger input FUNCTION_CALL_EVENT
function TOP  = fcn(interpolationMethod)
%#codegen
% Checks if the parameter satisfies dimensionality requirements
if(numel(interpolationMethod.Value) ~= 1)
   TranslateError('The parameter ''medusa_surround_db_interpolation'' must be single dimensional.'); 
end

% Checks if the parameter value follows bound requirements
if((interpolationMethod.Value ~= 0) && (interpolationMethod.Value ~= 1))
   TranslateError('The value of ''medusa_surround_db_interpolation'' must be either 0 (for linear interpolation) or 1 (for dB-linear interpolation).'); 
end

TOP = interpolationMethod.Value;

end

== matlab function Model_TranslationEngine64/ModelPreAmp/DecRate/Medusa5H1/MedusaHoligram/Medusa5H1 Part 3/On/Premix/Premix with Mono-Surround & CAE with Fade Ramper/SLC Tuning/Max Level CS/Trivial Translation ==
  data: TOP output size=[MedusaPremixConfig.CS_out MedusaPremixConfig.CS_in]; maxGain_CS input; MedusaPremixConfig parameter; TOP_CAE output size=[MedusaPremixConfig.CS_out MedusaPremixConfig.NumTailComp.CS]
  events: trigger input FUNCTION_CALL_EVENT
function [TOP, TOP_CAE] = fcn(maxGain_CS, MedusaPremixConfig)
%#codegen
numCSIn = MedusaPremixConfig.CS_in;
NumCAEWeights = MedusaPremixConfig.NumTailComp.CS;

NumRows = MedusaPremixConfig.CS_out;
NumColumns = numCSIn + NumCAEWeights;
if(~ MedusaPremixConfig.includeCAE)
    NumColumns = numCSIn;
end

% Checks if the parameter satisfies dimensionality requirements
if(maxGain_CS.Size(1) ~= NumRows || maxGain_CS.Size(2) ~= NumColumns)
    TranslateError('The parameter ''medusa_premix_cs_max'' must be a matrix consisting of %d rows and %d columns.', NumRows, NumColumns);
end

% Checks if the parameter values follow bound requirements
checkValues = (maxGain_CS.Value < 0);
if(sum(sum(checkValues)))          % Results in 0 if all values in the matrix respect the bound requirements
    TranslateError('The weights in ''medusa_premix_cs_max'' must be greater than or equal to 0.');
end

% Assigning the parameter values to respective tuneTOPS
TOP = maxGain_CS.Value(:, 1:numCSIn);
if(~ MedusaPremixConfig.includeCAE)
    TOP_CAE = zeros(NumRows, NumCAEWeights);
else
    TOP_CAE = maxGain_CS.Value(:, numCSIn+1:end);
end

end

== matlab function Model_TranslationEngine64/ModelPreAmp/DecRate/Medusa5H1/MedusaHoligram/Medusa5H1 Part 3/On/Premix/Premix with Mono-Surround & CAE with Fade Ramper/SLC Tuning/Max Level Left/Trivial Translation ==
  data: TOP output size=[MedusaPremixConfig.LR_out MedusaPremixConfig.LR_in]; maxGain_Left input; MedusaPremixConfig parameter; TOP_CAE output size=[MedusaPremixConfig.LR_out MedusaPremixConfig.NumTailComp.LR]
  events: trigger input FUNCTION_CALL_EVENT
function [TOP, TOP_CAE]  = fcn(maxGain_Left, MedusaPremixConfig)
%#codegen
numLRIn = MedusaPremixConfig.LR_in;
NumCAEWeights = MedusaPremixConfig.NumTailComp.LR;

NumRows = MedusaPremixConfig.LR_out;
NumColumns = numLRIn + NumCAEWeights;
if(~ MedusaPremixConfig.includeCAE)
    NumColumns = numLRIn;
end

% Checks if the parameter satisfies dimensionality requirements
if(maxGain_Left.Size(1) ~= NumRows || maxGain_Left.Size(2) ~= NumColumns)
    TranslateError('The parameter ''medusa_premix_left_max'' must be a matrix consisting of %d rows and %d columns.', NumRows, NumColumns);
end

% Checks if the parameter values follow bound requirements
checkValues = (maxGain_Left.Value < 0);
if(sum(sum(checkValues)))          % Results in 0 if all values in the matrix respect the bound requirements
    TranslateError('The weights in ''medusa_premix_left_max'' must be greater than or equal to 0.');
end

% Assigning the parameter values to respective tuneTOPS
TOP = maxGain_Left.Value(:, 1:numLRIn);
if(~ MedusaPremixConfig.includeCAE)
    TOP_CAE = zeros(NumRows, NumCAEWeights);
else
    TOP_CAE = maxGain_Left.Value(:, numLRIn+1:end);
end

end

== matlab function Model_TranslationEngine64/ModelPreAmp/DecRate/AudioPilot35/Audiopilot_3_5/GainCalculation/BoostMapAdjustment/AudiopilotOn/Bass1Enable ==
  data: on input; slopeOut output; slope input
  events: trigger input FUNCTION_CALL_EVENT
function slopeOut  = enable(on,slope)
%#codegen
slopeOut = slope.Value * on.Value;

== matlab function Model_TranslationEngine64/ModelPreAmp/DecRate/Medusa5H1/MedusaHoligram/Medusa5H1 Part 3/On/Premix/Premix with Mono-Surround & CAE with Fade Ramper/SLC Tuning/Max Level Right/Trivial Translation ==
  data: TOP output size=[MedusaPremixConfig.LR_out MedusaPremixConfig.LR_in]; maxGain_Right input; MedusaPremixConfig parameter; TOP_CAE output size=[MedusaPremixConfig.LR_out MedusaPremixConfig.NumTailComp.LR]
  events: trigger input FUNCTION_CALL_EVENT
function [TOP, TOP_CAE]  = fcn(maxGain_Right, MedusaPremixConfig)
%#codegen
numLRIn = MedusaPremixConfig.LR_in;
NumCAEWeights = MedusaPremixConfig.NumTailComp.LR;

NumRows = MedusaPremixConfig.LR_out;
NumColumns = numLRIn + NumCAEWeights;
if(~ MedusaPremixConfig.includeCAE)
    NumColumns = numLRIn;
end

% Checks if the parameter satisfies dimensionality requirements
if(maxGain_Right.Size(1) ~= NumRows || maxGain_Right.Size(2) ~= NumColumns)
    TranslateError('The parameter ''medusa_premix_right_max'' must be a matrix consisting of %d rows and %d columns.', NumRows, NumColumns);
end

% Checks if the parameter values follow bound requirements
checkValues = (maxGain_Right.Value < 0);
if(sum(sum(checkValues)))          % Results in 0 if all values in the matrix respect the bound requirements
    TranslateError('The weights in ''medusa_premix_right_max'' must be greater than or equal to 0.');
end

% Assigning the parameter values to respective tuneTOPS
TOP = maxGain_Right.Value(:, 1:numLRIn);
if(~ MedusaPremixConfig.includeCAE)
    TOP_CAE = zeros(NumRows, NumCAEWeights);
else
    TOP_CAE = maxGain_Right.Value(:, numLRIn+1:end);
end

end

== matlab function Model_TranslationEngine64/ModelPreAmp/DecRate/Medusa5H1/MedusaHoligram/Medusa5H1 Part 3/On/Premix/Premix with Mono-Surround & CAE with Fade Ramper/SLC Tuning/Min Level CS/Trivial Translation ==
  data: TOP output size=[MedusaPremixConfig.CS_out MedusaPremixConfig.CS_in]; minGain_CS input; MedusaPremixConfig parameter; TOP_CAE output size=[MedusaPremixConfig.CS_out MedusaPremixConfig.NumTailComp.CS]
  events: trigger input FUNCTION_CALL_EVENT
function [TOP, TOP_CAE]  = fcn(minGain_CS, MedusaPremixConfig)
%#codegen
numCSIn = MedusaPremixConfig.CS_in;
NumCAEWeights = MedusaPremixConfig.NumTailComp.CS;

NumRows = MedusaPremixConfig.CS_out;
NumColumns = numCSIn + NumCAEWeights;
if(~ MedusaPremixConfig.includeCAE)
    NumColumns = numCSIn;
end

% Checks if the parameter satisfies dimensionality requirements
if(minGain_CS.Size(1) ~= NumRows || minGain_CS.Size(2) ~= NumColumns)
    TranslateError('The parameter ''medusa_premix_cs_min'' must be a matrix consisting of %d rows and %d columns.', NumRows, NumColumns);
end

% Checks if the parameter values follow bound requirements
checkValues = (minGain_CS.Value < 0);
if(sum(sum(checkValues)))          % Results in 0 if all values in the matrix respect the bound requirements
    TranslateError('The weights in ''medusa_premix_cs_min'' must be greater than or equal to 0.');
end

% Assigning the parameter values to respective tuneTOPS
TOP = minGain_CS.Value(:, 1:numCSIn);
if(~ MedusaPremixConfig.includeCAE)
    TOP_CAE = zeros(NumRows, NumCAEWeights);
else
    TOP_CAE = minGain_CS.Value(:, numCSIn+1:end);
end

end

== matlab function Model_TranslationEngine64/ModelPreAmp/DecRate/Medusa5H1/MedusaHoligram/Medusa5H1 Part 3/On/Premix/Premix with Mono-Surround & CAE with Fade Ramper/SLC Tuning/Min Level Left/Trivial Translation ==
  data: TOP output size=[MedusaPremixConfig.LR_out MedusaPremixConfig.LR_in]; minGain_Left input; MedusaPremixConfig parameter; TOP_CAE output size=[MedusaPremixConfig.LR_out MedusaPremixConfig.NumTailComp.LR]
  events: trigger input FUNCTION_CALL_EVENT
function [TOP, TOP_CAE]  = fcn(minGain_Left, MedusaPremixConfig)
%#codegen
numLRIn = MedusaPremixConfig.LR_in;
NumCAEWeights = MedusaPremixConfig.NumTailComp.LR;

NumRows = MedusaPremixConfig.LR_out;
NumColumns = numLRIn + NumCAEWeights;
if(~ MedusaPremixConfig.includeCAE)
    NumColumns = numLRIn;
end

% Checks if the parameter satisfies dimensionality requirements
if(minGain_Left.Size(1) ~= NumRows || minGain_Left.Size(2) ~= NumColumns)
    TranslateError('The parameter ''medusa_premix_left_min'' must be a matrix consisting of %d rows and %d columns.', NumRows, NumColumns);
end

% Checks if the parameter values follow bound requirements
checkValues = (minGain_Left.Value < 0);
if(sum(sum(checkValues)))          % Results in 0 if all values in the matrix respect the bound requirements
    TranslateError('The weights in ''medusa_premix_left_min'' must be greater than or equal to 0.');
end

% Assigning the parameter values to respective tuneTOPS
TOP = minGain_Left.Value(:, 1:numLRIn);
if(~ MedusaPremixConfig.includeCAE)
    TOP_CAE = zeros(NumRows, NumCAEWeights);
else
    TOP_CAE = minGain_Left.Value(:, numLRIn+1:end);
end

end

== matlab function Model_TranslationEngine64/ModelPreAmp/DecRate/Medusa5H1/MedusaHoligram/Medusa5H1 Part 3/On/Premix/Premix with Mono-Surround & CAE with Fade Ramper/SLC Tuning/Min Level Right/Trivial Translation ==
  data: TOP output size=[MedusaPremixConfig.LR_out MedusaPremixConfig.LR_in]; minGain_Right input; MedusaPremixConfig parameter; TOP_CAE output size=[MedusaPremixConfig.LR_out MedusaPremixConfig.NumTailComp.LR]
  events: trigger input FUNCTION_CALL_EVENT
function [TOP, TOP_CAE]  = fcn(minGain_Right, MedusaPremixConfig)
%#codegen
numLRIn = MedusaPremixConfig.LR_in;
NumCAEWeights = MedusaPremixConfig.NumTailComp.LR;

NumRows = MedusaPremixConfig.LR_out;
NumColumns = numLRIn + NumCAEWeights;
if(~ MedusaPremixConfig.includeCAE)
    NumColumns = numLRIn;
end

% Checks if the parameter satisfies dimensionality requirements
if(minGain_Right.Size(1) ~= NumRows || minGain_Right.Size(2) ~= NumColumns)
    TranslateError('The parameter ''medusa_premix_right_min'' must be a matrix consisting of %d rows and %d columns.', NumRows, NumColumns);
end

% Checks if the parameter values follow bound requirements
checkValues = (minGain_Right.Value < 0);
if(sum(sum(checkValues)))          % Results in 0 if all values in the matrix respect the bound requirements
    TranslateError('The weights in ''medusa_premix_right_min'' must be greater than or equal to 0.');
end

% Assigning the parameter values to respective tuneTOPS
TOP = minGain_Right.Value(:, 1:numLRIn);
if(~ MedusaPremixConfig.includeCAE)
    TOP_CAE = zeros(NumRows, NumCAEWeights);
else
    TOP_CAE = minGain_Right.Value(:, numLRIn+1:end);
end

end

== matlab function Model_TranslationEngine64/ModelPreAmp/DecRate/AudioPilot35/Audiopilot_3_5/NoiseEstimationVariant/RegularNoiseEstimation/LFNoiseEstimatorCoh/EnergyLpfCoef/TimeConstant2Coefficient ==
  data: coef output; tau input; DecRate3 parameter
  events: trigger input FUNCTION_CALL_EVENT
function coef  = fcn(tau,DecRate3)
% Convert time constant to filter coefficient
%#codegen

wc = 1/(DecRate3*tau.Value);
coef = (1-sin(wc))/cos(wc);

== matlab function Model_TranslationEngine64/ModelPreAmp/DecRate/AudioPilot35/Audiopilot_3_5/GainCalculation/BoostMapAdjustment/AudiopilotOn/Midrange1Enable ==
  data: on input; slopeOut output; slope input
  events: trigger input FUNCTION_CALL_EVENT
function slopeOut  = enable(on,slope)
%#codegen
slopeOut = slope.Value * on.Value;

== matlab function Model_TranslationEngine64/ModelPreAmp/DecRate/AudioPilot35/Audiopilot_3_5/GainCalculation/BoostMapAdjustment/AudiopilotOn/Treble1Enable ==
  data: on input; slopeOut output; slope input
  events: trigger input FUNCTION_CALL_EVENT
function slopeOut  = enable(on,slope)
%#codegen
slopeOut = slope.Value * on.Value;
